simulink model "modelo2"  (Simulink 7.9)
settings: Solver=ode4  StartTime=0.0  StopTime=t_final  FixedStep=t_step  RelTol=1e-3
InitFcn:
  | modelo2Initialization
values from neighbouring files (symbols this model uses):
  t_step = 0.05    [Quadrotor_Simualtion.m]    (also in modelo2Initialization.m = 0.01)
undefined symbols (not defined in the file or in its folder): Earth, IC, sigbuilder_block, WGS84
libraries: simulink_extras x2, aerolibfltsims x2, aerolibtransform2 x1, aerolibanimutils x1
settings Model: Creator=claus  LastModifiedBy=claus  SimulationMode=accelerator
settings SolverCC: ShapePreserveControl=EnableAll
settings OptimizationCC: SimCompilerOptimization=On  AccelVerboseBuild=on
settings ModelReferenceCC: EnableParallelModelReferenceBuilds=on

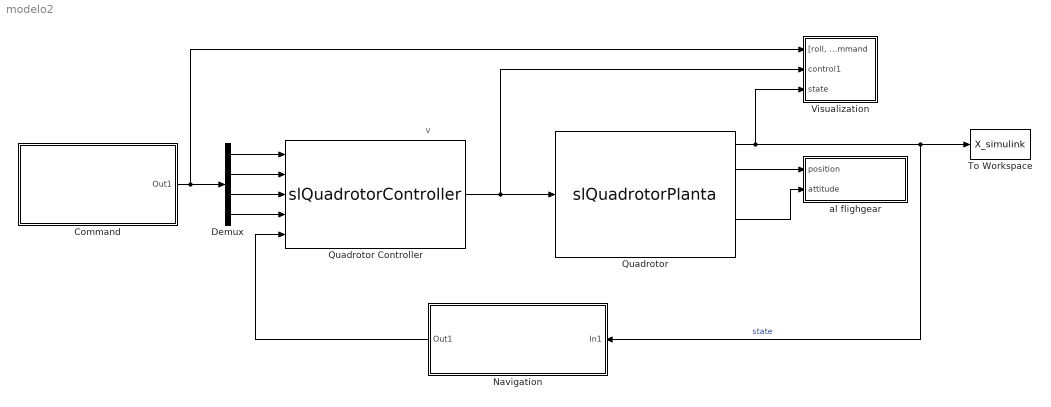
== system modelo2 ==
  note: v
  Command : Subsystem
      mask Display:
      | fprintf('Command \n \n')
      | port_label('output', 1, '[roll, pitch, yaw, height]')
  Demux : Demux
  Navigation : Subsystem
  Quadrotor : M-S-Function  FunctionName=slQuadrotorPlanta
      mask init:
      | slQuadrotorPlantaInitialization
      mask Display:
      | port_label('output', 1, 'state x(1:12)')
      | port_label('output', 2, 'pos (I)')
      | port_label('output', 3, 'vel (B)')
      | port_label('output', 4, 'Euler (I) [Roll Pitch Yaw]')
      | port_label('output', 5, '\omega (B)')
      | port_label('input', 1, 'Control [f1 f2 f3 f4]')
  Quadrotor Controller : M-S-Function  FunctionName=slQuadrotorController
      mask Display:
      | port_label('output', 1, 'control\n [f1 f2 f3 f4]')
      | port_label('input', 1, 'roll command')
      | port_label('input', 2, 'pitch command')
      | port_label('input', 3, 'yaw command')
      | port_label('input', 4, 'altitude command')
      | port_label('input', 5, 'state')
  To Workspace : ToWorkspace  VariableName=X_simulink  SampleTime=-1  SaveFormat=Timeseries
  Visualization : Subsystem
  al flighgear : Subsystem
  wires:
  Quadrotor Controller/1 -> Quadrotor/1, Visualization/2(control1)
  Quadrotor/1 -> Visualization/3(state), To Workspace/1, Navigation/1(In1)  "state"
  Quadrotor/2 -> al flighgear/1(position)
  Quadrotor/4 -> al flighgear/2(attitude)
  Command/1(Out1) -> Demux/1, Visualization/1("[roll, pitch, yaw, height] command")
  Navigation/1(Out1) -> Quadrotor Controller/5
  Demux/1 -> Quadrotor Controller/1
  Demux/2 -> Quadrotor Controller/2
  Demux/3 -> Quadrotor Controller/3
  Demux/4 -> Quadrotor Controller/4

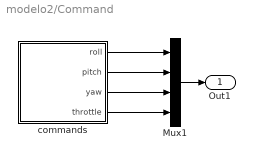
== system modelo2/Command ==
  Mux1 : Mux
  commands : Subsystem  Tag=STV Subsys  LoadFcn=sigbuilder_block('load',[407 4 616 433 ]);  StartFcn=sigbuilder_block('start');  StopFcn=sigbuilder_block('stop');  ClipboardFcn=sigbuilder_block('clipboard');  mask(Sigbuilder block){}
      mask help: Simulink:masks:SigbuilderBlock_MD
      mask init:
      | if ~strcmp(get_param(bdroot(gcbh),'SimulationStatus'),'stopped') tuvar = sigbuilder_block('maskInit'); end
      settings: CopyFcn=sigbuilder_block('copy');  DeleteFcn=sigbuilder_block('delete');  ModelCloseFcn=sigbuilder_block('modelClose');  PreSaveFcn=sigbuilder_block('preSave');  PauseFcn=sigbuilder_block('pause');  ContinueFcn=sigbuilder_block('continue');  NameChangeFcn=sigbuilder_block('namechange');  OpenFcn=sigbuilder_block('open',[409 13 615 433 ]);  CloseFcn=sigbuilder_block('close');
      mask Display: plot(0, 0, 100, 100,[2, 2, 32, 32, 2], [68, 8, 8, 68, 68],[32, 2], [38, 38], [32, 19, 2],[53, 60, 44], [32, 17, 17, 2],[16, 16, 31, 31]);txt = getActiveGroup(gcbh);text(2, 100, txt,'verticalAlignment', 'top');
  Out1 : Outport
  wires:
  commands/1(roll) -> Mux1/1
  commands/2(pitch) -> Mux1/2
  commands/3(yaw) -> Mux1/3
  commands/4(throttle) -> Mux1/4
  Mux1/1 -> Out1/1

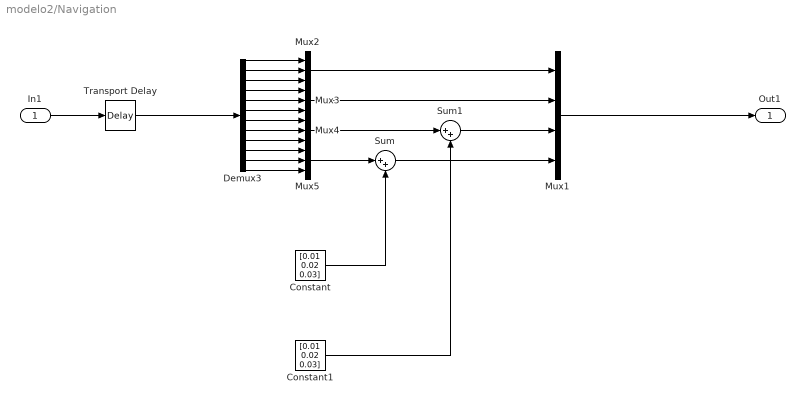
== system modelo2/Navigation ==
  In1 : Inport
  Constant : Constant  Value=[0.01 0.02 0.03]
  Constant1 : Constant  Value=[0.01 0.02 0.03]
  Demux3 : Demux  Outputs=12
  Mux1 : Mux
  Mux{2..5} (4 alike) : Mux  Inputs=3
  Sum : Sum  Inputs=|++
  Sum1 : Sum  Inputs=|++
  Transport Delay : TransportDelay  DelayTime=t_step*1
  Out1 : Outport
  wires:
  In1/1 -> Transport Delay/1
  Demux3/1 -> Mux2/1
  Demux3/2 -> Mux2/2
  Demux3/3 -> Mux2/3
  Demux3/4 -> Mux3/1
  Demux3/5 -> Mux3/2
  Demux3/6 -> Mux3/3
  Demux3/7 -> Mux4/1
  Demux3/8 -> Mux4/2
  Demux3/9 -> Mux4/3
  Demux3/10 -> Mux5/1
  Demux3/11 -> Mux5/2
  Demux3/12 -> Mux5/3
  Mux2/1 -> Mux1/1
  Transport Delay/1 -> Demux3/1
  Mux3/1 -> Mux1/2
  Mux4/1 -> Sum1/1
  Mux5/1 -> Sum/1
  Sum1/1 -> Mux1/3
  Sum/1 -> Mux1/4
  Constant/1 -> Sum/2
  Constant1/1 -> Sum1/2
  Mux1/1 -> Out1/1

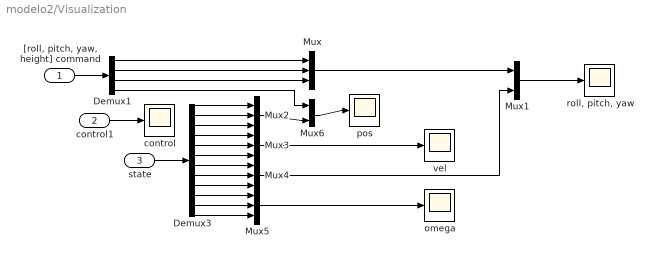
== system modelo2/Visualization ==
  "[roll, pitch, yaw, height] command" : Inport
  control1 : Inport  Port=2
  state : Inport  Port=3
  Demux1 : Demux
  Demux3 : Demux  Outputs=12
  Mux{,2..5} (5 alike) : Mux  Inputs=3
  Mux1 : Mux  Inputs=2
  Mux6 : Mux  Inputs=2
  control : Scope
      settings: YMin=5.55112e-17  YMax=1
  omega : Scope
      settings: YMin=-7  SaveName=ScopeData3
  pos : Scope
      settings: YMin=-15  YMax=40  SaveName=ScopeData2
  "roll, pitch, yaw" : Scope
      settings: YMin=-1  YMax=7
  vel : Scope
      settings: YMin=-12.5  YMax=7.5  SaveName=ScopeData4
  wires:
  Demux1/1 -> Mux/1
  Demux1/2 -> Mux/2
  Demux1/3 -> Mux/3
  Mux/1 -> Mux1/1
  Mux1/1 -> "roll, pitch, yaw"/1
  Demux3/1 -> Mux2/1
  Demux3/2 -> Mux2/2
  Demux3/3 -> Mux2/3
  Demux3/4 -> Mux3/1
  Demux3/5 -> Mux3/2
  Demux3/6 -> Mux3/3
  Demux3/7 -> Mux4/1
  Demux3/8 -> Mux4/2
  Demux3/9 -> Mux4/3
  Demux3/10 -> Mux5/1
  Demux3/11 -> Mux5/2
  Demux3/12 -> Mux5/3
  Mux4/1 -> Mux1/2
  Mux6/1 -> pos/1
  Demux1/4 -> Mux6/1
  Mux2/1 -> Mux6/2
  Mux5/1 -> omega/1
  Mux3/1 -> vel/1
  "[roll, pitch, yaw, height] command"/1 -> Demux1/1
  control1/1 -> control/1
  state/1 -> Demux3/1

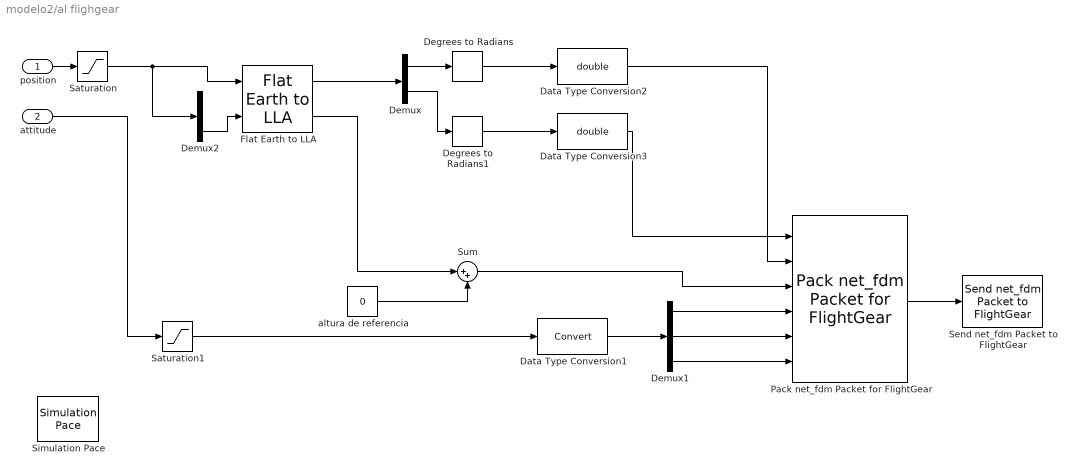
== system modelo2/al flighgear ==
  position : Inport
  attitude : Inport  Port=2
  Data Type Conversion1 : DataTypeConversion
  Data Type Conversion2 : DataTypeConversion  OutDataTypeStr=double
  Data Type Conversion3 : DataTypeConversion  OutDataTypeStr=double
  Degrees to Radians : simulink_extras/Transformations/Degrees to Radians
  Degrees to Radians1 : simulink_extras/Transformations/Degrees to Radians
  Demux : Demux  Outputs=2
  Demux1 : Demux  Outputs=3
  Demux2 : Demux  Outputs=3
  Flat Earth to LLA : aerolibtransform2/Flat Earth to LLA  units=Metric (MKS)  ptype=Earth (WGS84)  F=1/298.257223563  R=6378137  LL0=IC.LatLonAltOnEarth(1:2)  psi=0
  Pack net_fdm Packet for FlightGear : aerolibfltsims/Pack net_fdm Packet for FlightGear  FlightGearVersion=v2.0  ShowPositionAttitudeInputs=on  ShowVelocityAccelerationInputs=off  ShowControlSurfacePositionInputs=off  ShowEngineFuelInputs=off  ShowLandingGearInputs=off  ShowEnvironmentInputs=off  SampleTime=-1
  Saturation : Saturate  UpperLimit=100  LowerLimit=-100
  Saturation1 : Saturate  UpperLimit=100  LowerLimit=-100
  Send net_fdm Packet to FlightGear : aerolibfltsims/Send net_fdm Packet to FlightGear  DestinationIpAddress=10.0.3.203  DestinationPort=5502  LocalIpPort=-1  varLen=off  SampleTime=-1
  Simulation Pace : aerolibanimutils/Simulation Pace  SimulationPace=1  SleepMode=MATLAB Thread  OutputPaceError=off  SampleTime=-1
      settings: AttributesFormatString=%<SimulationPace> sec/sec
  Sum : Sum  Inputs=|++
  altura de referencia : Constant  Value=0
  wires:
  position/1 -> Saturation/1
  attitude/1 -> Saturation1/1
  Pack net_fdm Packet for FlightGear/1 -> Send net_fdm Packet to FlightGear/1
  Demux1/1 -> Pack net_fdm Packet for FlightGear/4
  Demux1/2 -> Pack net_fdm Packet for FlightGear/5
  Demux1/3 -> Pack net_fdm Packet for FlightGear/6
  Data Type Conversion1/1 -> Demux1/1
  Flat Earth to LLA/1 -> Demux/1
  Demux2/3 -> Flat Earth to LLA/2
  Degrees to Radians/1 -> Data Type Conversion2/1
  Degrees to Radians1/1 -> Data Type Conversion3/1
  Demux/1 -> Degrees to Radians/1
  Demux/2 -> Degrees to Radians1/1
  Data Type Conversion3/1 -> Pack net_fdm Packet for FlightGear/1
  Data Type Conversion2/1 -> Pack net_fdm Packet for FlightGear/2
  Flat Earth to LLA/2 -> Sum/1
  altura de referencia/1 -> Sum/2
  Sum/1 -> Pack net_fdm Packet for FlightGear/3
  Saturation/1 -> Demux2/1, Flat Earth to LLA/1
  Saturation1/1 -> Data Type Conversion1/1

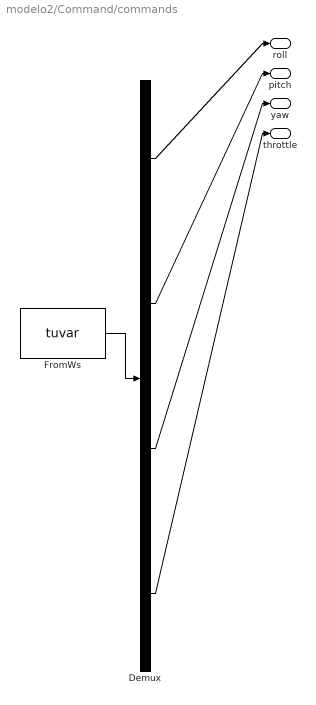
== system modelo2/Command/commands ==
  Demux : Demux  Tag=STV Demux
  FromWs : FromWorkspace  Tag=STV FromWs  VariableName=tuvar  SampleTime=0  SigBuilderData=DataTag0  VnvData=DataTag1
      SigBuilderData=|
      | common.afterFinalStr = 'Extrapolate'
      | common.sampleTime = 0
      | dataSet.timeRange = [0 15]
      | dataSet.name = 'Group 1'
      | sbobj.Groups.Name = 'Group 1'
      | sbobj.Groups.Signals(1).Name = 'roll'
      | sbobj.Groups.Signals(1).XData = [0 5 6.5 9 10.05 15]
      | sbobj.Groups.Signals(1).YData = [0 0 6.28318530718 6.28318530718 0 0]
      | sbobj.Groups.Signals(2).Name = 'pitch'
      | sbobj.Groups.Signals(2).XData = [0 0.8 1 1.4 3.5 5 11.4 15]
      | sbobj.Groups.Signals(2).YData = [0 0 0 -0.4 -0.4 0 0 0]
      | sbobj.Groups.Signals(3).Name = 'yaw'
      | sbobj.Groups.Signals(3).XData = [0 0.6 3.45 5 6.5 8.5 15]
      | sbobj.Groups.Signals(3).YData = [0 0 0 0 0 0 0]
      | sbobj.Groups.Signals(4).Name = 'throttle'
      | sbobj.Groups.Signals(4).XData = [0 6 6 9.35 9.35 15]
      | sbobj.Groups.Signals(4).YData = [-6 -15 -8.4 -8.4 -1.6 -1.6]
      | sbobj.Groups.TimeRange = [0 15]
  roll : Outport  Tag=STV Outport
  pitch : Outport  Tag=STV Outport  Port=2
  yaw : Outport  Tag=STV Outport  Port=3
  throttle : Outport  Tag=STV Outport  Port=4
  wires:
  FromWs/1 -> Demux/1
  Demux/1 -> roll/1
  Demux/2 -> pitch/1
  Demux/3 -> yaw/1
  Demux/4 -> throttle/1
